simulink model "test"  (R2020a)
settings: Solver=VariableStepAuto  StartTime=0.0  StopTime=100000  RelTol=1e-3
settings Model: Creator=prans  LastModifiedBy=prans

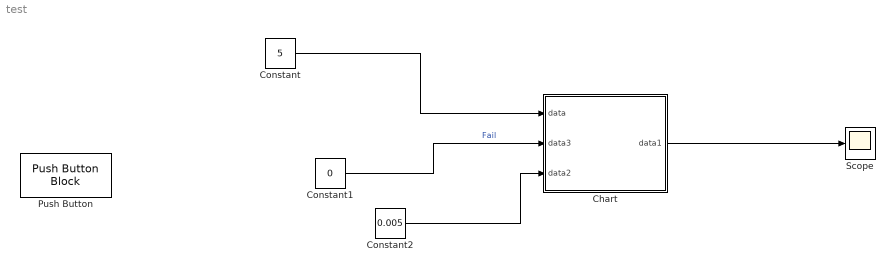
== system test ==
  Chart : Stateflow chart  TreatAsAtomicUnit=on
  Constant : Constant  Value=5
  Constant1 : Constant  Value=0
  Constant2 : Constant  Value=0.005
  Push Button : PushButtonBlock
  Scope : Scope
  wires:
  Constant/1 -> Chart/1(data)
  Chart/1(data1) -> Scope/1
  Constant1/1 -> Chart/2(data3)  "Fail"
  Constant2/1 -> Chart/3(data2)

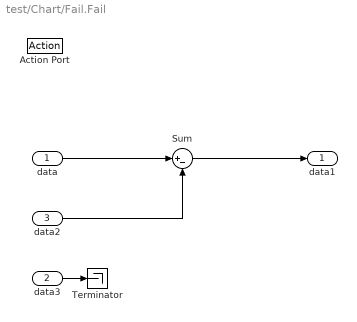
== system test/Chart/Fail.Fail ==
  data : Inport
  data3 : Inport  Port=2
  data2 : Inport  Port=3
  Action Port : ActionPort
      settings: CopyFcn=Stateflow.SLINSF.SimulinkMan.removeBlockPreDeleteFcn  PreDeleteFcn=Stateflow.SLINSF.SimulinkMan.unsafePredeleteFcn
  Sum : Sum  Inputs=|+-
  Terminator : Terminator
  data1 : Outport
  wires:
  data/1 -> Sum/1
  data2/1 -> Sum/2
  Sum/1 -> data1/1
  data3/1 -> Terminator/1

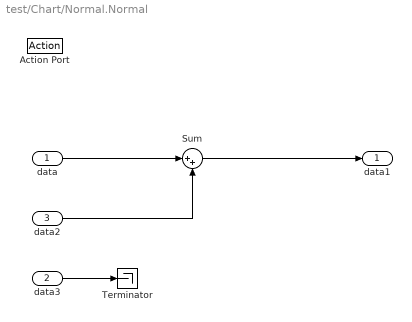
== system test/Chart/Normal.Normal ==
  data : Inport
  data3 : Inport  Port=2
  data2 : Inport  Port=3
  Action Port : ActionPort
      settings: CopyFcn=Stateflow.SLINSF.SimulinkMan.removeBlockPreDeleteFcn  PreDeleteFcn=Stateflow.SLINSF.SimulinkMan.unsafePredeleteFcn
  Sum : Sum  Inputs=|++
  Terminator : Terminator
  data1 : Outport
  wires:
  data2/1 -> Sum/2
  data/1 -> Sum/1
  Sum/1 -> data1/1
  data3/1 -> Terminator/1

== stateflow chart test/Chart ==
  state Fail
    state Fail
    (default) -> Fail.Fail
  state Normal
    state Normal
    (default) -> Normal.Normal
  (default) -> Normal
  Fail -> Normal : [data3 == 1]
  Normal -> Fail : [data3 == 0]
  data: sf_internal_action_state_placeholder_data local double size=1 =0; sf_internal_action_state_placeholder_data local double size=1 =0; data input; data3 input; data1 output; data2 input
